simulink model "project"  (R2020a)
settings: Solver=FixedStepAuto  StartTime=0.0  StopTime=inf  FixedStep=0.001  RelTol=1e-3
libraries: simulink x1
settings Model: EnablePacing=on  Creator=Main  LastModifiedBy=Main
settings SolverCC: ZeroCrossAlgorithm=Adaptive
settings DebuggingCC: IgnoredZcDiagnostic=none
settings ConfigComp: DVTestSuiteOptimization=Auto  DVDetectOutOfBounds=on

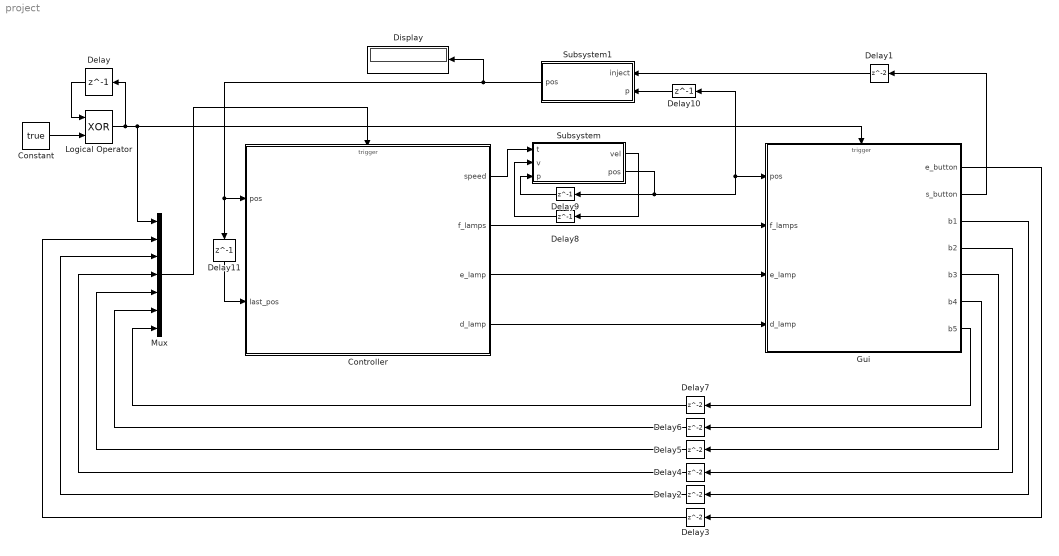
== system project ==
  Constant : Constant  Value=true  OutDataTypeStr=boolean
  Controller : Stateflow chart  TreatAsAtomicUnit=on
  Delay : Delay  DelayLength=1
  Delay{1..7} (7 alike) : Delay
  Delay10 : Delay  DelayLength=1  InitialCondition=1
  Delay11 : Delay  DelayLength=1
  Delay8 : Delay  DelayLength=1
  Delay9 : Delay  DelayLength=1  InitialCondition=1
  Display : Display
  Gui : Stateflow chart  TreatAsAtomicUnit=on
  Logical Operator : Logic  Operator=XOR  AllPortsSameDT=off  OutDataTypeStr=boolean
  Mux : Mux  Inputs=7
  Subsystem : Subsystem
  Subsystem1 : Subsystem
  wires:
  Controller/3(e_lamp) -> Gui/3(e_lamp)
  Controller/4(d_lamp) -> Gui/4(d_lamp)
  Controller/2(f_lamps) -> Gui/2(f_lamps)
  Logical Operator/1 -> Gui/Trigger, Mux/1, Delay/1
  Mux/1 -> Controller/Trigger
  Gui/1(e_button) -> Delay3/1
  Delay3/1 -> Mux/2
  Delay2/1 -> Mux/3
  Gui/3(b1) -> Delay2/1
  Gui/4(b2) -> Delay4/1
  Gui/5(b3) -> Delay5/1
  Gui/6(b4) -> Delay6/1
  Delay4/1 -> Mux/4
  Delay5/1 -> Mux/5
  Delay6/1 -> Mux/6
  Delay7/1 -> Mux/7
  Gui/7(b5) -> Delay7/1
  Constant/1 -> Logical Operator/2
  Delay/1 -> Logical Operator/1
  Controller/1(speed) -> Subsystem/1(t)
  Subsystem/2(pos) -> Delay10/1, Gui/1(pos), Delay9/1
  Delay8/1 -> Subsystem/2(v)
  Subsystem/1(vel) -> Delay8/1
  Delay9/1 -> Subsystem/3(p)
  Delay11/1 -> Controller/2(last_pos)
  Gui/2(s_button) -> Delay1/1
  Delay10/1 -> Subsystem1/2(p)
  Subsystem1/1(pos) -> Display/1, Controller/1(pos), Delay11/1
  Delay1/1 -> Subsystem1/1(inject)

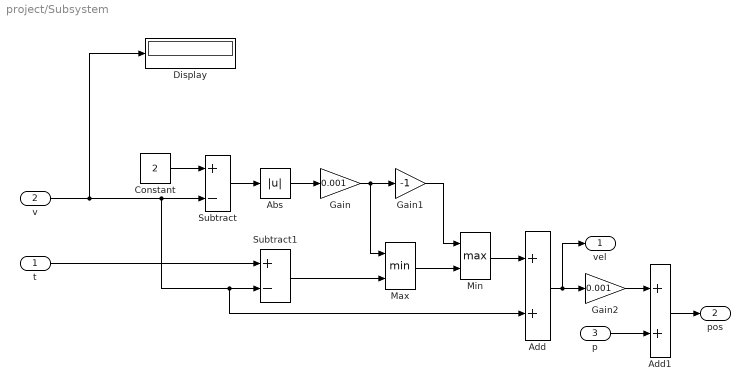
== system project/Subsystem ==
  t : Inport
  v : Inport  Port=2
  p : Inport  Port=3
  Abs : Abs
  Add : Sum
  Add1 : Sum
  Constant : Constant  Value=2
  Display : Display
  Gain : Gain  Gain=0.001
  Gain1 : Gain  Gain=-1
  Gain2 : Gain  Gain=0.001
  Max : MinMax  Inputs=2
  Min : MinMax  Function=max  Inputs=2
  Subtract : Sum  Inputs=+-
  Subtract1 : Sum  Inputs=+-
  vel : Outport
  pos : Outport  Port=2
  wires:
  v/1 -> Display/1, Add/2, Subtract1/2, Subtract/2
  Subtract/1 -> Abs/1
  Abs/1 -> Gain/1
  t/1 -> Subtract1/1
  Subtract1/1 -> Max/2
  Gain/1 -> Gain1/1, Max/1
  Max/1 -> Min/2
  Gain1/1 -> Min/1
  Min/1 -> Add/1
  Add/1 -> vel/1, Gain2/1
  Gain2/1 -> Add1/1
  p/1 -> Add1/2
  Add1/1 -> pos/1
  Constant/1 -> Subtract/1

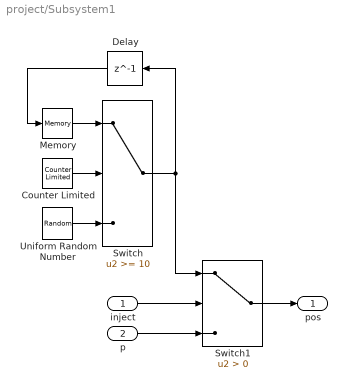
== system project/Subsystem1 ==
  inject : Inport
  p : Inport  Port=2
  Counter Limited : simulink/Sources/Counter Limited  uplimit=1000  tsamp=-1
  Delay : Delay  DelayLength=1
  Memory : Memory
  Switch : Switch  Threshold=10
  Switch1 : Switch  Criteria=u2 > Threshold
  Uniform Random Number : UniformRandomNumber  Minimum=0  Maximum=5  SampleTime=0.001
  pos : Outport
  wires:
  Counter Limited/1 -> Switch/2
  Memory/1 -> Switch/1
  Switch/1 -> Switch1/1, Delay/1
  Delay/1 -> Memory/1
  inject/1 -> Switch1/2
  Switch1/1 -> pos/1
  p/1 -> Switch1/3
  Uniform Random Number/1 -> Switch/3

== stateflow chart project/Gui ==
  settings: sampleTime=0.01  executeAtInitialization=1
  state Gui
    en: ml.mk_figure(); ml.mk_controls();
    du:
    ml.set_lights(f_lamps, d_lamp, e_lamp);
    ml.move_lift(pos);
    state Button4 [parallel]
      settings: executionOrder=4
      state On
        en: b4 = 1;
      state Off
        en: b4 = 0;
      (default) -> Gui.Button4.Off
      Gui.Button4.Off -> Gui.Button4.On : [ml.get_state(4)]
      Gui.Button4.On -> Gui.Button4.Off : [f_lamps[3] > 0]
          | /{ml.set_state(4,0);}
    state Button5 [parallel]
      settings: executionOrder=8
      state On
        en: b5 = 1;
      state Off
        en: b5 = 0;
      (default) -> Gui.Button5.Off
      Gui.Button5.Off -> Gui.Button5.On : [ml.get_state(5)]
      Gui.Button5.On -> Gui.Button5.Off : [f_lamps[4] > 0]
          | /{ml.set_state(5,0);}
    state Button3 [parallel]
      settings: executionOrder=3
      state On
        en: b3 = 1;
      state Off
        en: b3 = 0;
      (default) -> Gui.Button3.Off
      Gui.Button3.Off -> Gui.Button3.On : [ml.get_state(3)]
      Gui.Button3.On -> Gui.Button3.Off : [f_lamps[2] > 0]
          | /{ml.set_state(3,0);}
    state Doors [parallel]
      settings: executionOrder=7
      state On
        en: ml.set_door(1);
      state Closed
        en: ml.set_door(0);
      (default) -> Closed
      Closed -> Gui.Doors.On : [d_lamp == 1]
      Gui.Doors.On -> Closed : [d_lamp == 0]
    state Button2 [parallel]
      settings: executionOrder=2
      state On
        en: b2 = 1;
      state Off
        en: b2 = 0;
      (default) -> Gui.Button2.Off
      Gui.Button2.Off -> Gui.Button2.On : [ml.get_state(2)]
      Gui.Button2.On -> Gui.Button2.Off : [f_lamps[1] > 0]
          | /{ml.set_state(2,0);}
    state ButtonS [parallel]
      settings: executionOrder=6
      state On
        en: s_button = 1;
        ml.inject(1);
      state Off
        en: s_button = 0;
        ml.inject(0);
      (default) -> Gui.ButtonS.Off
      Gui.ButtonS.Off -> Gui.ButtonS.On : [ml.get_state(ST)]
          | {ml.set_state(ST,0);}
      Gui.ButtonS.On -> Gui.ButtonS.Off : [ml.get_state(ST)]
          | {ml.set_state(ST,0);}
    state Button1 [parallel]
      settings: executionOrder=1
      state On
        en: b1 = 1;
      state Off
        en: b1 = 0;
      (default) -> Gui.Button1.Off
      Gui.Button1.Off -> Gui.Button1.On : [ml.get_state(1)]
      Gui.Button1.On -> Gui.Button1.Off : [f_lamps[0] > 0]
          | /{ml.set_state(1,0);}
    state ButtonE [parallel]
      settings: executionOrder=5
      state On
        en: e_button = 1;
      state Off
        en: e_button = 0;
      (default) -> Gui.ButtonE.Off
      Gui.ButtonE.Off -> Gui.ButtonE.On : [ml.get_state(EM)]
          | /{last_estate = e_lamp;}
      Gui.ButtonE.On -> Gui.ButtonE.Off : [e_lamp != last_estate || after(1, sec)]
          | /{ml.set_state(EM,0);}
  data: pos input double; f_lamps input int8 size=5; e_lamp input boolean; d_lamp input boolean; e_button output boolean; s_button output boolean; EM constant double =6; ST constant double =7; b1 output boolean =0; b2 output boolean =0; b3 output boolean =0; b4 output boolean =0; b5 output boolean =0; last_estate local double =1
  events: TIC input RISING_EDGE_EVENT

== stateflow chart project/Controller ==
  settings: sampleTime=0.01  executeAtInitialization=1
  state ControlModule
    state FloorButton [parallel]
      settings: executionOrder=2
      state Buttons
      Buttons -> Buttons [order 1] : B1 /{lamp_state(1); Button}
      (default) -> Buttons
      Buttons -> Buttons [order 5] : B5 /{lamp_state(5);
          |        Button}
      Buttons -> Buttons [order 2] : B2 /{lamp_state(2);
          |         Button}
      Buttons -> Buttons [order 3] : B3 /{lamp_state(3); Button}
      Buttons -> Buttons [order 4] : B4 /{lamp_state(4);
          |         Button}
    state Controller [parallel]
      settings: executionOrder=1
      state Normal
        state Moving
          state FullSpeed
          state Break
            du: speed = target - pos;
          (default) -> FullSpeed
          FullSpeed -> Break [order 1] : [ab(pos - target) < 0.4]
        state Idle
          en: speed = 0;
        state Plan
          en:
          plan();
          speed = direction * MAX_SPEED;
        state Doors
          en:
          f_lamps[target-1] = LAMP_HERE;
          d_lamp = 1;
        state DoorWait
        Idle -> Plan [order 3] : [sumlamps() > 0]
        (default) -> Idle
        Plan -> Moving [order 2] : [at_floor() != target]
        Idle -> Plan [order 1] : Button
        FullSpeed -> Plan [order 2] : Button
        Plan -> Idle [order 1] : [target < 1]
        Idle -> Doors [order 2] : [d_lamp]
        Doors -> Plan : [after(5, sec)]
            | /{d_lamp = 0;
            |   f_lamps[target-1] = LAMP_OFF;}
        Plan -> Doors [order 3] : [at_floor() == target && speed == 0]
        Moving -> DoorWait : [at_floor() == target]
            | /{speed = 0;}
        DoorWait -> Doors : [after(0.5,sec)]
      state Emergency
        en:
        e_lamp = 1;
        speed = 0;
        state WaitForRelease
        state Stabilize
        Stabilize -> WaitForRelease [order 2] : [after(5, sec)]
        Stabilize -> Stabilize [order 1] : [ab(pos - last_pos) > POS_FAULT]
        WaitForRelease -> Stabilize [order 1] : [ab(pos - last_pos) > POS_FAULT]
      (default) -> Normal
      WaitForRelease -> Doors [order 2] : Emergency[d_lamp == 1]
          | /{e_lamp = 0;}
      WaitForRelease -> Normal [order 3] : Emergency[d_lamp == 0]
          | /{e_lamp = 0;}
      Normal -> WaitForRelease [order 1] : Emergency
      Normal -> Stabilize [order 2] : [ab(pos - last_pos) > POS_FAULT]
  (default) -> ControlModule
  data: y function_output double; k function_input double; s function_output int8; v function_output double; x function_input double; speed output double; pos input double; f_lamps output int8 size=5; e_lamp output boolean; LAMP_OFF constant int8 =0; LAMP_ON constant int8 =1; LAMP_TARGET constant int8 =2; LAMP_HERE constant int8 =3; MAX_SPEED constant double =1; target local int8 =-1; direction local double =0; d_lamp output boolean; FLOORS constant int8 =5; last_pos input; POS_FAULT constant double =0.1
  events: TIC input RISING_EDGE_EVENT; Emergency input RISING_EDGE_EVENT; B1 input RISING_EDGE_EVENT; B2 input RISING_EDGE_EVENT; B3 input RISING_EDGE_EVENT; B4 input RISING_EDGE_EVENT; Button local RISING_EDGE_EVENT; B5 input RISING_EDGE_EVENT
  function y = at_floor:
    | % calculate which floor the elevator is on
    | % if elevator not at a floor, return -1
    | function y = at_floor()
    |     %y = -1;
    |     %for k = 1:FLOORS
    |     %    if abs(pos - k) < 0.01
    |     %        y = k;
    |     %        return;
    |     %    end
    |     nearest = round(pos);
    |     if abs(pos - nearest) < 0.02
    |         y = nearest;
    |     else
    |         y = -1;
    |     end
    | end
  function plan:
    | % set target of elevator, and update the floor state
    | % since the lamps colour is based on floor state, why not use that?
    | function plan()
    |     old_target = target;    % used to set state of old target from Target to On
    |     % if currently going up, prioritise the up direction
    |     if direction > 0
    |         if look_up(old_target)
    |             % nothing up, look down
    |             if look_down(old_target)
    |                 % nothing down either, elevator is idle
    |                 direction = 0;
    |                 target = int8(-1);
    |             end
    |         end
    |     else
    |         % if going down, or if idle, look down first then up
    |         if look_down(old_target)
    |             if look_up(old_target)
    |                 % noting, elevator is idle
    |                 direction = 0;
    |                 target = int8(-1);
    |             end
    |         end
    |     end
    | end
    | 
    | % look floors above
    | % if no target, returns 1 - otherwise returns 0
    | function no = look_up(old_target)
    |     % just in case elevator is slightly above top floor
    |     % shouldn't happen, but just in case
    |     next_floor = min(ceil(pos+0.5), FLOORS);
    |     no = 1;
    |     % look at above floors, starting with nearest
    |     for k = next_floor:FLOORS
    |         % if floor light is on, or if floor is already target
    |         if f_lamps(k) == LAMP_ON || f_lamps(k) == LAMP_TARGET
    |             % if not target, old target should not be target
    |             % but should still be on
    |             if old_target > 0
    |                 if f_lamps(old_target) == LAMP_TARGET
    |                     f_lamps(old_target) = LAMP_ON;
    |                 end
    |             end
    |             % set as target
    |             f_lamps(k) = LAMP_TARGET;
    |             target = int8(k);
    |             if target ~= at_floor()
    |                 direction = 1;
    |             end
    |             no = 0;
    |             return;
    |         end
    |     end
    | end
    | 
    | % look floors below
    | % if no target, returns 1 - otherwise returns 0
    | function no = look_down(old_target)
    |     % just in case elevator is slightly below bottom floor
    |     % shouldn't happen, but just in case
    |     next_floor = max(floor(pos-0.5), 1);
    |     no = 1;
    |     % look at below floors, starting with nearest
    |     for k = 1:next_floor
    |         ind = int8(next_floor + 1 - k);
    |         % if floor light is on, or if floor is already target
    |         if f_lamps(ind) == LAMP_ON || f_lamps(ind) == LAMP_TARGET
    |             % if not target, old target should not be target
    |             % but should still be on
    |             if old_target > 0
    |                 if f_lamps(old_target) == LAMP_TARGET
    |                     f_lamps(old_target) = LAMP_ON;
    |                 end
    |             end
    |             % set as target
    |             f_lamps(ind) = LAMP_TARGET;
    |             target = ind;
    |             if target ~= at_floor()
    |                 direction = -1;
    |             end
    |             no = 0;
    |             return;
    |         end
    |     end
    | end
  function lamp_state(k):
    | % toggle state of lamp k between on and off
    | % ignored if lamp is in state target or here
    | function lamp_state(k)
    |     %for k=1:FLOORS
    |         if f_lamps(k) == LAMP_OFF
    |             f_lamps(k) = LAMP_ON;
    |         end
    |     %end
    | end
  function s = sumlamps:
    | function s = sumlamps()
    |     s = f_lamps(1) + f_lamps(2) + f_lamps(3) + f_lamps(4) + f_lamps(5);
    | end
  function v = ab(x):
    | function v = ab(x)
    |     v = abs(x);
    | end
